simulink model "AVR_H_inf_LMI_nonlinear_"  (R2022a)
settings: Solver=VariableStepAuto  StartTime=0.0  StopTime=120  RelTol=1e-3
undefined symbols (not defined in the file or in its folder): D1, Delta
libraries: spsThreePhaseParallelRLCLoadLib x2, spsLoadFlowBusLib x2, spsThreePhaseSourceLib x1, spsThreePhaseFaultLib x1, spsExcitationSystemLib x1, spsHydraulicTurbineandGovernorLib x1, spsThreePhaseTransformerTwoWindingsLib x1, spsVoltageMeasurementLib x1, spsGroundLib x1, spspowerguiLib x1, spsSynchronousMachinepuStandardLib x1
settings Model: Creator=asus  LastModifiedBy=asus

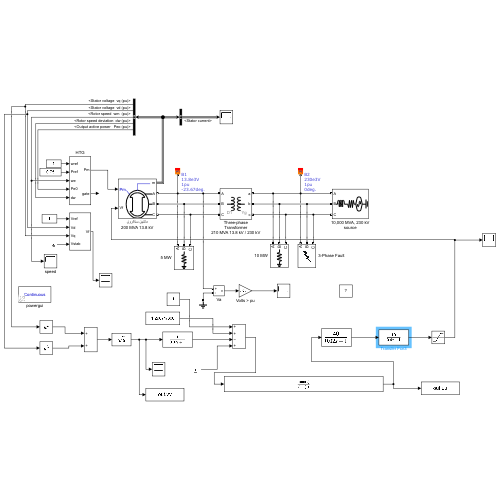
[thumbnail: Simulink's stored preview of the top-level diagram]
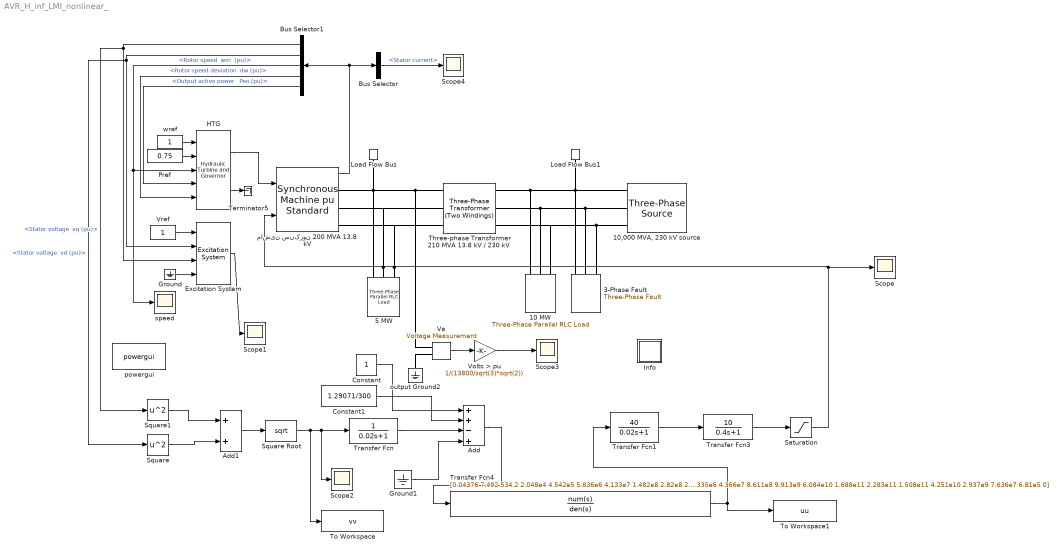
== system AVR_H_inf_LMI_nonlinear_ ==
  10 MW : spsThreePhaseParallelRLCLoadLib/Three-Phase Parallel RLC Load  LConnTagsString=A|B|C  Configuration=Y (grounded)  NominalVoltage=230e3  Vabc=[1e3 1e3 1e3]  Vabcp=[1e3 1e3 1e3]  NominalFrequency=60  UnbalancedPower=off  ActivePower=10000000  InductivePower=0  CapacitivePower=0  Pabc=[10e3 9e3 11e3]  QLabc=[100 90 110]  QCabc=[100 90 110]  Pabcp=[10e3 9e3 11e3]  QLabcp=[100 90 110]  QCabcp=[100 90 110]  Measurements=None  LoadType=constant Z
  "10,000 MVA, 230 kV source" : spsThreePhaseSourceLib/Three-Phase Source  InternalConnection=Yg  VoltagePhases=off  Voltage=(230000)*1.00006  PhaseAngle=-0.77547  Voltage_phases=[25e3 25e3 25e3]/sqrt(3)  PhaseAngles_phases=[0 -120 +120]  Frequency=60  NonIdealSource=on  SpecifyImpedance=on  Resistance=0.529  Inductance=0.0140  ShortCircuitLevel=10000e6  BaseVoltage=230e3  XRratio=10  BusType=swing  Pref=0  Qref=0  Prefabc=[10e3, 10e3, 10e3]  Qrefabc=[0, 0, 0]  Qmin=-Inf  Qmax=Inf
  3-Phase Fault : spsThreePhaseFaultLib/Three-Phase Fault  InitialStates=0  FaultA=on  FaultB=on  FaultC=on  GroundFault=on  SwitchTimes=[ 0.1 0.2]  External=off  SwitchStatus=NaN  FaultResistance=1e-3  GroundResistance=1e-3  SnubberResistance=inf  SnubberCapacitance=inf  Measurements=None
  5 MW : spsThreePhaseParallelRLCLoadLib/Three-Phase Parallel RLC Load  LConnTagsString=A|B|C  Configuration=Y (grounded)  NominalVoltage=13.8e3  Vabc=[1e3 1e3 1e3]  Vabcp=[1e3 1e3 1e3]  NominalFrequency=60  UnbalancedPower=off  ActivePower=5000000  InductivePower=0  CapacitivePower=0  Pabc=[10e3 9e3 11e3]  QLabc=[100 90 110]  QCabc=[100 90 110]  Pabcp=[10e3 9e3 11e3]  QLabcp=[100 90 110]  QCabcp=[100 90 110]  Measurements=None  LoadType=constant Z
  Add : Sum  Inputs=++-+
  Add1 : Sum
  Bus Selector : BusSelector  OutputSignals=Stator current
  Bus Selector1 : BusSelector  OutputSignals="dq0 components.Stator voltage  vq (pu),dq0 components.Stator voltage  vd (pu),Mechanical.Rotor speed  wm  (pu),Mechanical.Rotor speed deviation  dw (pu),Output active power   Peo (pu)"
  Constant : Constant
  Constant1 : Constant  Value=1.29071/300
  Excitation System : spsExcitationSystemLib/Excitation System  tr=20e-3  reg=[ 300, 0.001 ]  exc=[ 1, 0 ]  tgr=[ 0, 0 ]  damp=[ 0.001, 0.1 ]  sat=[ 0, 0 ]  lim=[ -11.5, 11.5, 0 ]  v0=[1,1.29071]
      settings: SourceProductBaseCode=PS
  Ground : Ground
  Ground1 : Ground
  HTG : spsHydraulicTurbineandGovernorLib/Hydraulic Turbine and Governor  sm="[ 10/3  0.07 ]"  gate="[  0.01  0.97518  -0.1  0.1 ]"  reg="[  0.05  1.163  0.105  0  0.01  ]"  hyd="[  0  2.67  ]"  dref=0  po=0.751606
      settings: SourceProductBaseCode=PS
  Info : Subsystem
      settings: OpenFcn=showdemo(bdroot(gcb))
      mask Display: disp('?')
  Load Flow Bus : spsLoadFlowBusLib/Load Flow Bus  LConnTagsString=a  Phases=single  Connectors=on one side  ID=B1  Vbase=13.8e3  Vref=1  Vangle=0  VLF=1  VLFb=1  VLFc=1  angleLF=-23.67  angleLFb=0  angleLFc=0
      settings: AttributesFormatString=%<ID>\n%<Vbase>V\n%<VLF>pu\n%<angleLF>deg.  SourceProductBaseCode=PS
  Load Flow Bus1 : spsLoadFlowBusLib/Load Flow Bus  LConnTagsString=a  Phases=single  Connectors=on one side  ID=B2  Vbase=230e3  Vref=1  Vangle=0  VLF=1  VLFb=1  VLFc=1  angleLF=0  angleLFb=0  angleLFc=0
      settings: AttributesFormatString=%<ID>\n%<Vbase>V\n%<VLF>pu\n%<angleLF>deg.  SourceProductBaseCode=PS
  Pref : Constant  Value=0.75
  Saturation : Saturate  UpperLimit=11.5  LowerLimit=-11.5
  Scope{,1..4} (5 alike) : Scope
  Square : Math  Operator=square
  Square Root : Sqrt
  Square1 : Math  Operator=square
  Terminator5 : Terminator
  Three-phase Transformer 210 MVA 13.8 kV / 230 kV : spsThreePhaseTransformerTwoWindingsLib/Three-Phase Transformer (Two Windings)  Winding1Connection=Delta (D1)  Winding2Connection=Yg  CoreType=Three single-phase transformers  SetSaturation=off  Hysteresis=off  DataFile='hysteresis'  SetInitialFlux=off  Measurements=None  UNITS=pu  NominalPower=[ 210e6 60 ]  Winding1="[ 13.8e3 0.0027  0.08]"  Winding2=[ 230e3 0.0027 0.08]  Rm=500  Lm=500  L0=0.5  Saturation="[ 0,0  ;  0.005,1.2  ;  1.0,1.4 ]"  InitialFluxes=[ 0.8 , -0.8 , 0.7 ]  BreakLoop=off  DiscreteSolver=Trapezoidal iterative  DataType=off  TransfoNumber=0
  To Workspace : ToWorkspace  VariableName=vv  SaveFormat=Timeseries  SampleTime=-1
  To Workspace1 : ToWorkspace  VariableName=uu  SaveFormat=Timeseries  SampleTime=-1
  Transfer Fcn : TransferFcn  Denominator=[0.02 1]
  Transfer Fcn1 : TransferFcn  Numerator=[40]  Denominator=[0.02 1]
  Transfer Fcn3 : TransferFcn  Numerator=[10]  Denominator=[0.4 1]
  Transfer Fcn4 : TransferFcn  Numerator=[0.04376 7.492 534.2 2.048e4 4.542e5 5.836e6 4.133e7 1.482e8 2.82e8 2.905e8 1.552e8 3.685e7 2.257e6 5.292e4 430.3]  Denominator=[1 240.1 2.423e4 1.335e6 4.366e7 8.611e8 9.913e9 6.084e10 1.688e11 2.283e11 1.508e11 4.251e10 2.937e9 7.636e7 6.81e5 0]
  Va : spsVoltageMeasurementLib/Voltage Measurement  Tag=PoWeRsYsTeMmEaSuReMeNt  PhasorSimulation=off  OutputType=Magnitude  PSBequivalent=0
  Volts > pu : Gain  Gain=1/(13800/sqrt(3)*sqrt(2))  SaturateOnIntegerOverflow=on  OutDataTypeStr=Inherit: Same as input  ParamDataTypeStr=Inherit: Same as input
  Vref : Constant
  output Ground2 : spsGroundLib/Ground  LConnTagsString=a
  powergui : spspowerguiLib/powergui  Priority=2  SimulationMode=Continuous  SampleTime=0  frequency=60  Iterations=50  frequencyindice=60  Pbase=100e6  ErrMax=0.0001  UnitsV=kV  UnitsW=MW  buscounter=0  FunctionMessages=off  echomessages=off  EnableUseOfTLC=off  CurrentSourceSwitches=off  DisableSnubberDevices=off  DisableRonSwitches=off  DisableVfSwitches=off  DisplayEquations=off  AutomaticDiscreteSolvers=off  SolverType=Tustin  Interpol=off  ExternalGateDelay=off  methode=off  Ts=0  x0status=blocks  SPID=on  SwTol=0  HookPort=off  NonlinearTolerance=1e-4  nMaxIteration=100  ContinueOnMaxIteration=off  RestoreLinks=warning  ResistiveCurrentMeasurement=off  Frange=logspace(0,3,50)  Ylog=off  Xlog=off  ShowGrid=off  save=off  variable=ZData  structure=0  ZoomFFT=on  StartTime=0.0  cycles=2  DisplayStyle=off  fundamental=60  FreqAxis=off  MaxFrequency=1000  frequencyindicesteady=1  RmsSteady=1  display=off
  speed : Scope
  wref : Constant
  ماشین سنکرون 200 MVA 13.8 kV : spsSynchronousMachinepuStandardLib/Synchronous Machine pu Standard  PresetModel=No  MechanicalLoad=Mechanical power Pm  ShowDetailedParameters=on  RotorType=Salient-pole  Units=per unit standard parameters  MeasurementBus=off  NominalParameters="[ 200E6  13800   60 ]"  Reactances1=[ 31 32 33 34 35 36 37 ]  Reactances2=[ 1.305, 0.296, 0.252, 0.474, 0.243, 0.18 ]  dAxisTimeConstants=Short-circuit  qAxisTimeConstants=Short-circuit  TimeConstants1=[]  TimeConstants2=[]  TimeConstants3=[]  TimeConstants4=[]  TimeConstants5=[ 1.01, 0.053, 0.1 ]  TimeConstants6=[]  TimeConstants7=[ 1.01, 0.053, 0.1 ]  TimeConstants8=[]  StatorResistance=2.8544e-3  Mechanical=[ 3.2 0 2]  PolePairs=2  InitialConditions=[0 -94.2826 0.750185 0.750185 0.750185 -24.943 -144.943 95.057 1.29071]  SetSaturation=off  Saturation=[0.6404,0.7127,0.8441,0.9214,0.9956,1.082,1.19,1.316,1.457;0.7,0.7698,0.8872,0.9466,0.9969,1.046,1.1,1.151,1.201]  LoadFlowParameters=[1 150000000 0 0]  TsPowergui=0  TsBlock=-1  IterativeModel=Trapezoidal non iterative  IterativeDiscreteModel=Trapezoidal non iterative  BusType=PV  Pref=150000000  Qref=0  Qmin=-Inf  Qmax=Inf  PLF=0  QLF=0
      settings: SourceProductBaseCode=PS
  wires:
  Ground1/1 -> Add/4
  Add1/1 -> Square Root/1
  Bus Selector1/4 -> HTG/5  "<Rotor speed deviation  dw (pu)>"
  HTG/1 -> ماشین سنکرون 200 MVA 13.8 kV/1
  Pref/1 -> HTG/2
  Bus Selector1/3 -> speed/1, HTG/3  "<Rotor speed  wm  (pu)>"
  Volts > pu/1 -> Scope3/1
  Bus Selector1/5 -> HTG/4  "<Output active power   Peo (pu)>"
  Transfer Fcn1/1 -> Transfer Fcn3/1
  Vref/1 -> Excitation System/1
  Constant/1 -> Add/1
  Square/1 -> Add1/2
  Bus Selector1/2 -> Square/1, Excitation System/2  "<Stator voltage  vd (pu)>"
  wref/1 -> HTG/1
  Transfer Fcn/1 -> Add/3
  Square1/1 -> Add1/1
  Constant1/1 -> Add/2
  Square Root/1 -> To Workspace/1, Scope2/1, Transfer Fcn/1
  ماشین سنکرون 200 MVA 13.8 kV/1 -> Bus Selector/1, Bus Selector1/1
  Transfer Fcn3/1 -> Saturation/1
  Excitation System/1 -> Scope1/1
  Ground/1 -> Excitation System/4
  Saturation/1 -> ماشین سنکرون 200 MVA 13.8 kV/2, Scope/1
  Bus Selector/1 -> Scope4/1  "<Stator current>"
  HTG/2 -> Terminator5/1
  Va/1 -> Volts > pu/1
  Bus Selector1/1 -> Square1/1, Excitation System/3  "<Stator voltage  vq (pu)>"
  Add/1 -> Transfer Fcn4/1
  Transfer Fcn4/1 -> Transfer Fcn1/1, To Workspace1/1
  connections:
  Three-phase Transformer 210 MVA 13.8 kV / 230 kV/RConn1 -- 10 MW/LConn1 -- 3-Phase Fault/LConn1 -- "10,000 MVA, 230 kV source"/RConn1 -- Load Flow Bus1/LConn1
  Three-phase Transformer 210 MVA 13.8 kV / 230 kV/RConn2 -- 10 MW/LConn2 -- 3-Phase Fault/LConn2 -- "10,000 MVA, 230 kV source"/RConn2
  5 MW/LConn1 -- Load Flow Bus/LConn1 -- ماشین سنکرون 200 MVA 13.8 kV/RConn1 -- Three-phase Transformer 210 MVA 13.8 kV / 230 kV/LConn1 -- Va/LConn1
  3-Phase Fault/LConn3 -- "10,000 MVA, 230 kV source"/RConn3 -- Three-phase Transformer 210 MVA 13.8 kV / 230 kV/RConn3 -- 10 MW/LConn3
  5 MW/LConn2 -- Three-phase Transformer 210 MVA 13.8 kV / 230 kV/LConn2 -- ماشین سنکرون 200 MVA 13.8 kV/RConn2
  5 MW/LConn3 -- Three-phase Transformer 210 MVA 13.8 kV / 230 kV/LConn3 -- ماشین سنکرون 200 MVA 13.8 kV/RConn3
  output Ground2/LConn1 -- Va/LConn2

== system AVR_H_inf_LMI_nonlinear_/Info ==
